simulink model "Exercitiul1"  (R2016a)
settings: Solver=VariableStepDiscrete  StartTime=0.0  StopTime=100  RelTol=1e-3
undefined symbols (not defined in the file): entity, f, m, n
settings Model: Creator=Cristina  LastModifiedBy=Cristina

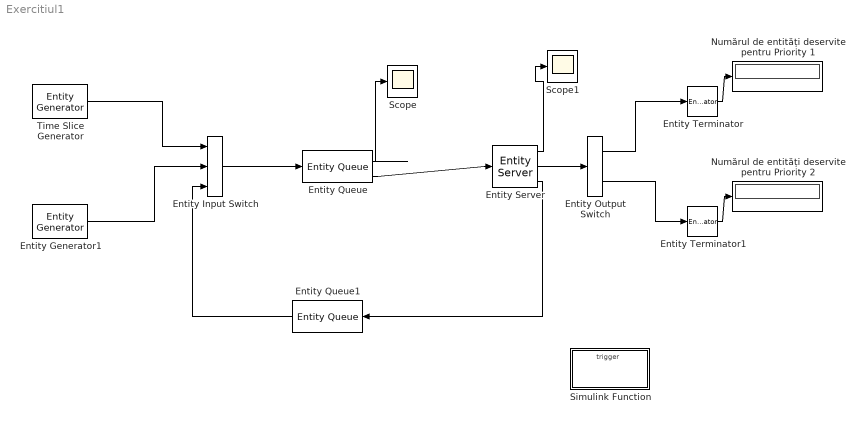
== system Exercitiul1 ==
  Entity Input Switch : EntityInputSwitch  InputPortMessageModes=m,m,m  OutputPortMessageModes=m  NumberInputPorts=3
      settings: InputPortMap=u1,u2,u3
  Entity Output Switch : EntityOutputSwitch  InputPortMessageModes=m  OutputPortMessageModes=m,m  SwitchingCriterion=From attribute  SwitchAttributeName=Priority
  Entity Generator1 : EntityGenerator  OutputPortMessageModes=m  TimeSource=MATLAB action  IntergenerationTimeAction=dt = exprnd(0.2);  AttributeName=Priority|ServiceTime|Preempted  AttributeInitialValue=2|0.18|0  EntityType=Structured  EntityTypeName=Entity
  Entity Queue : EntityQueue  InputPortMessageModes=m  OutputPortMessageModes=n,m  Capacity=50  QueueType=Priority  PrioritySource=Priority  NumberEntitiesInBlock=on
      settings: OutputPortMap=o1,o5
  Entity Queue1 : EntityQueue  InputPortMessageModes=m  OutputPortMessageModes=m  Capacity=50
      settings: OutputPortMap=o5
  Entity Server : EntityServer  InputPortMessageModes=m  OutputPortMessageModes=n,m,m  Capacity=1  ServiceTimeSource=Attribute  ExitAction=f(entity.Preempted);  PreemptAction=entity.Preempted = entity.Preempted +1;  PermitPreemptionBasedOnAttribute=on  SortingAttributeName=Priority  WriteResidualTimeToAttribute=on  ResidualTimeAttributeName=ServiceTime  Utilization=on
      settings: OutputPortMap=o5,o9,o10
  Entity Terminator : EntityTerminator  InputPortMessageModes=m  NumberEntitiesArrived=on
      settings: OutputPortMap=o0
  Entity Terminator1 : EntityTerminator  InputPortMessageModes=m  NumberEntitiesArrived=on
      settings: OutputPortMap=o0
  Numărul de entități deservite pentru Priority 1 : Display
  Numărul de entități deservite pentru Priority 2 : Display
  Scope : Scope
  Scope1 : Scope
  Simulink Function : Subsystem  TreatAsAtomicUnit=on
  Time Slice Generator : EntityGenerator  OutputPortMessageModes=m  Period=0.01  AttributeName=Priority|ServiceTime|Preempted  AttributeInitialValue=1|0|0  EntityType=Structured  EntityTypeName=Entity
  wires:
  Entity Input Switch/1 -> Entity Queue/1
  Entity Queue/2 -> Entity Server/1
  Time Slice Generator/1 -> Entity Input Switch/1
  Entity Generator1/1 -> Entity Input Switch/2
  Entity Queue/1 -> Scope/1
  Entity Server/1 -> Scope1/1
  Entity Server/3 -> Entity Queue1/1
  Entity Queue1/1 -> Entity Input Switch/3
  Entity Server/2 -> Entity Output Switch/1
  Entity Output Switch/1 -> Entity Terminator/1
  Entity Output Switch/2 -> Entity Terminator1/1
  Entity Terminator/1 -> Numărul de entități deservite pentru Priority 1/1
  Entity Terminator1/1 -> Numărul de entități deservite pentru Priority 2/1

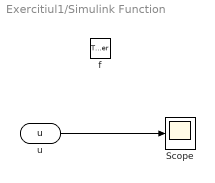
== system Exercitiul1/Simulink Function ==
  f : TriggerPort  TriggerType=function-call  IsSimulinkFunction=on  FunctionName=f  VariantControl=Variant
  Scope : Scope
  u : ArgIn  DisableCoverage=on  ArgumentName=u
  wires:
  u/1 -> Scope/1
